simulink model "Fuzzy_and_EKF_tightly"  (R2021b)
settings: Solver=ode4  StartTime=0.0  StopTime=200  FixedStep=1e-2  RelTol=1e-3
values from neighbouring files (symbols this model uses):
  n_J = 0.6    [sensors_model.m]
  n_W = 0.18    [sensors_model.m]
undefined symbols (not defined in the file or in its folder): measure
libraries: fuzblock x1
settings Model: Creator=francescoiotti  LastModifiedBy=pierg
settings ModelReferenceCC: ModelReferenceMinAlgLoopOccurrences=on

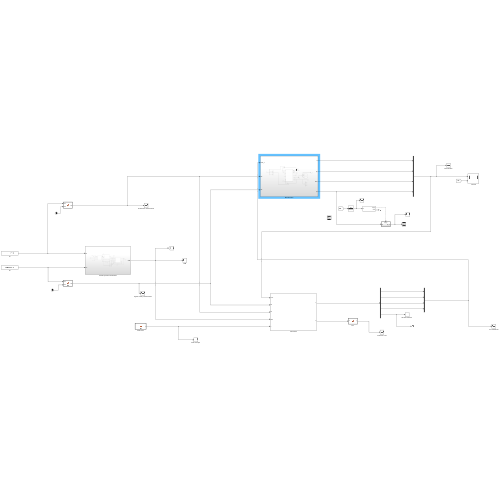
[thumbnail: Simulink's stored preview of the top-level diagram]
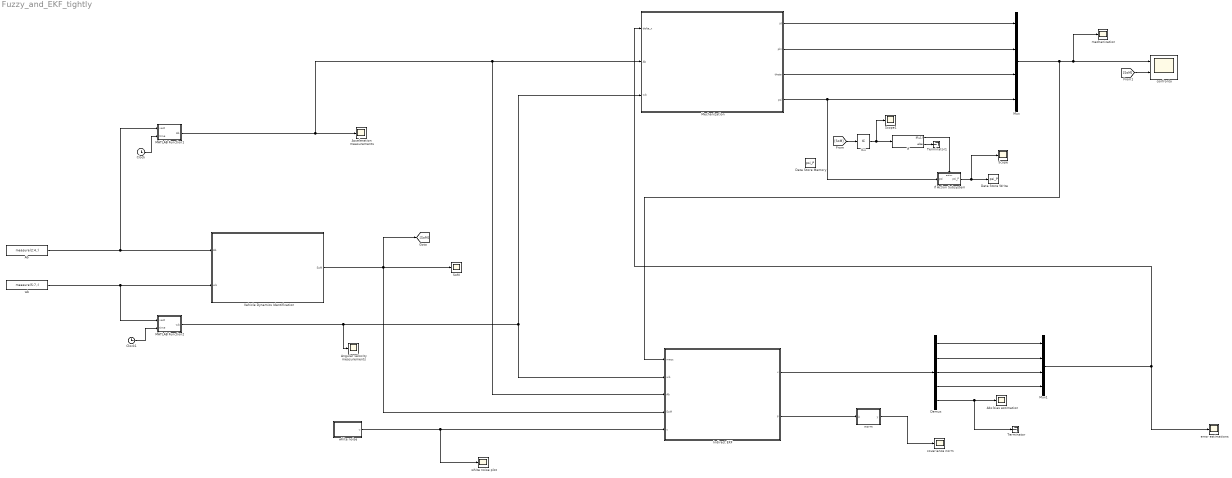
== system Fuzzy_and_EKF_tightly ==
  Ab : Constant  Value=measure(2:4,:)
  Abx bias estimation : Scope
  Acceleration measurements : Scope
  Angular velocity measurements : Scope
  Clock : Clock
  Clock1 : Clock
  Data Store Memory : DataStoreMemory  DataStoreName=psi_P  ReadBeforeWriteMsg=warning  WriteAfterWriteMsg=warning  WriteAfterReadMsg=warning  InitialValue=pi/2  ShowAdditionalParam=off
  Data Store Write : DataStoreWrite  DataStoreName=psi_P  IndexOptions=Index vector (dialog)  Indices=1  OutputSizes=1
  Demux : Demux  Outputs=5
  IC1 : InitialCondition
  If : If  IfExpression=u1
  If Action Subsystem : Subsystem  TreatAsAtomicUnit=on
  Indirect EKF : Subsystem
  MATLAB Function1 : MATLAB Function  TreatAsAtomicUnit=on
  MATLAB Function2 : MATLAB Function  TreatAsAtomicUnit=on
  Mechanization : Subsystem
  Mux : Mux
  Mux1 : Mux
  Scope : Scope
  Scope1 : Scope
  SoM : Scope
  Terminator : Terminator
  Terminator1 : Terminator
  Vehicle Dynamics Identification : Subsystem
  confronto : Scope  NumInputPorts=2
  covariance norm : Scope
  error estimations : Scope
  mechanization : Scope
  norm : MATLAB Function  TreatAsAtomicUnit=on
  wb : Constant  Value=measure(5:7,:)
  white noise : MATLAB Function  TreatAsAtomicUnit=on
  white noise plot : Scope
  wires:
  Vehicle Dynamics Identification/1(SoM) -> SoM/1, [SoM], Indirect EKF/4(SoM)
  Ab/1 -> MATLAB Function1/1(vect), Vehicle Dynamics Identification/1(Ab)
  Indirect EKF/2(P) -> norm/1(A)
  white noise/1(u) -> white noise plot/1, Indirect EKF/5(u)
  norm/1(y) -> covariance norm/1
  MATLAB Function1/1(Ab) -> Acceleration measurements/1, Indirect EKF/3(Ab), Mechanization/2(Ab)
  wb/1 -> MATLAB Function2/1(vect), Vehicle Dynamics Identification/2(wb)
  MATLAB Function2/1(wb) -> Angular velocity measurements/1, Mechanization/3(wb), Indirect EKF/2(wb)
  Clock/1 -> MATLAB Function1/2(time)
  Clock1/1 -> MATLAB Function2/2(time)
  Mux/1 -> confronto/1, mechanization/1, Indirect EKF/1(mecc)
  Mechanization/1(Vf) -> Mux/1
  Mechanization/2(phi) -> Mux/2
  Mechanization/3(theta) -> Mux/3
  Indirect EKF/1(x) -> Demux/1
  Demux/1 -> Mux1/1
  Demux/2 -> Mux1/2
  Demux/3 -> Mux1/3
  Demux/4 -> Mux1/4
  Mux1/1 -> Mechanization/1(delta_x), error estimations/1
  Demux/5 -> Abx bias estimation/1, Terminator/1
  If/1 -> If Action Subsystem/Action
  If Action Subsystem/1(psi_P) -> Scope/1, Data Store Write/1
  If/2 -> Terminator1/1
  [SoM] -> confronto/2
  Mechanization/4(psi) -> Mux/4, If Action Subsystem/1(psi)
  [SoM] -> IC1/1
  IC1/1 -> Scope1/1, If/1

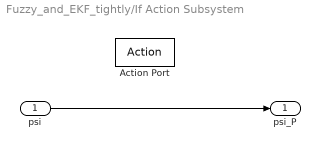
== system Fuzzy_and_EKF_tightly/If Action Subsystem ==
  psi : Inport
  Action Port : ActionPort  ActionPortLabel=if(u1)
  psi_P : Outport
  wires:
  psi/1 -> psi_P/1

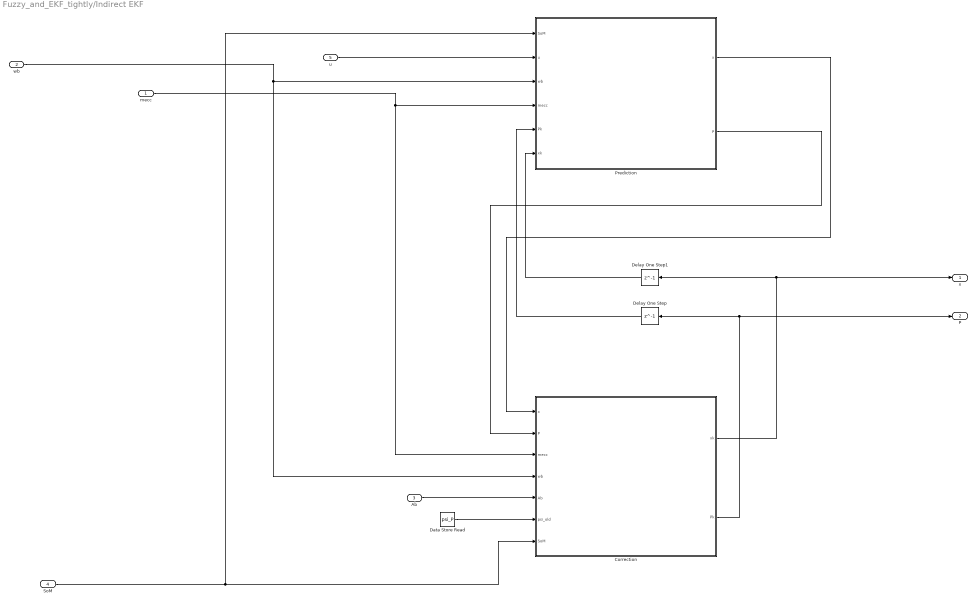
== system Fuzzy_and_EKF_tightly/Indirect EKF ==
  mecc : Inport
  wb : Inport  Port=2
  Ab : Inport  Port=3
  SoM : Inport  Port=4
  u : Inport  Port=5
  Correction : MATLAB Function  TreatAsAtomicUnit=on
  Data Store Read : DataStoreRead  DataStoreName=psi_P  IndexOptions=Index vector (dialog)  Indices=1  OutputSizes=1
  Delay One Step : Delay  DelayLength=1  InitialCondition=eye(5)
  Delay One Step1 : Delay  DelayLength=1  InitialCondition=[0 0 0 0 0]'
  Prediction : MATLAB Function  TreatAsAtomicUnit=on
  x : Outport
  P : Outport  Port=2
  wires:
  Prediction/1(x) -> Correction/1(x)
  Correction/1(xk) -> Delay One Step1/1, x/1
  Correction/2(Pk) -> Delay One Step/1, P/1
  Prediction/2(P) -> Correction/2(P)
  Delay One Step/1 -> Prediction/5(Pk)
  Delay One Step1/1 -> Prediction/6(xk)
  u/1 -> Prediction/2(u)
  wb/1 -> Correction/4(wb), Prediction/3(wb)
  Ab/1 -> Correction/5(Ab)
  mecc/1 -> Correction/3(mecc), Prediction/4(mecc)
  Data Store Read/1 -> Correction/6(psi_old)
  SoM/1 -> Correction/7(SoM), Prediction/1(SoM)

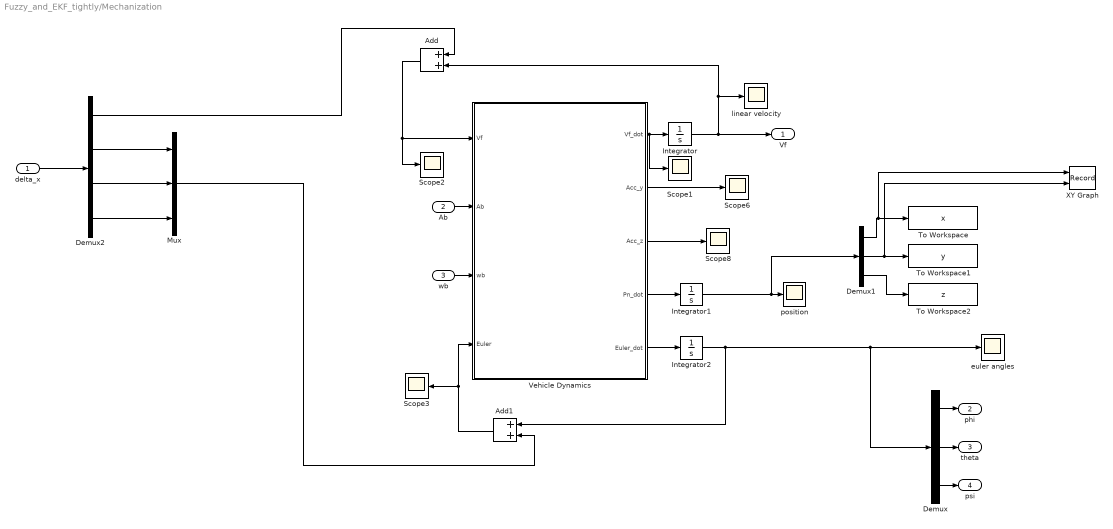
== system Fuzzy_and_EKF_tightly/Mechanization ==
  delta_x : Inport
  Ab : Inport  Port=2
  wb : Inport  Port=3
  Add : Sum
  Add1 : Sum
  Demux : Demux  Outputs=3
  Demux1 : Demux  Outputs=3
  Demux2 : Demux
  Integrator : Integrator
  Integrator1 : Integrator  InitialCondition=[0 0 0]'
  Integrator2 : Integrator  InitialCondition=[0 0 pi/2]'
  Mux : Mux  Inputs=3
  Scope{1..3,6,8} (5 alike) : Scope
  To Workspace : ToWorkspace  VariableName=x  SaveFormat=Structure  SampleTime=-1
  To Workspace1 : ToWorkspace  VariableName=y  SaveFormat=Structure  SampleTime=-1
  To Workspace2 : ToWorkspace  VariableName=z  SaveFormat=Structure  SampleTime=-1
  Vehicle Dynamics : MATLAB Function  TreatAsAtomicUnit=on
  XY Graph : Record  FileSettingsInternal="{\"entries\":[{\"content\":{\"excelSettings\":{\"content\":{},\"type\":\"Streamout.ExcelSettings\"}},\"type\":\"Streamout.FileSettingStorage\",\"uuid\":\"3c158775-b6e3-428c-9659-72c20ea76644\"}],\"packageUris\":[\"http://schema.mathworks.com/mf0/streamout_blocks/R2020a\"],\"version\":\"1.0\"}"  Layout=[1 1]  SignalsInternal="{\"entries\":[{\"content\":{\"signals\":[{\"content\":{\"blockPath\":[\"Fuzzy_and_EKF_tightly/Mechanization/XY Graph\"],\"channel\":[],\"dimensions\":[1,1],\"domain\":\"Fuzzy_and_EKF_tightly/Mechanization/XY Graph\",\"lineColor\":\"#edb120\",\"plots\":[],\"port\":1,\"sid\":[\"\"],\"signalID\":16325,\"signalName\":\"Demux1:1\"},\"type\":\"RecordBlkView.Signal\",\"uuid\":\"bfe6afe1-6902-4355-a286-55c02540e738\"},{\"content\":{\"blockPath\":[\"Fuzzy_and_EKF_tightly/Mechanization/XY Graph\"],\"channel\":[],\"dimensions\":[1,1],\"domain\":\"Fuzzy_and_EKF_tightly/Mechanization/XY Graph\",\"lineColor\":\"#7e2f8e\",\"plots\":[],\"port\":2,\"sid\":[\"\"],\"signalID\":16329,\"signalName\":\"Demux1:2\"},\"type\":\"RecordBlkView.Signal\",\"uuid\":\"bf2d8db9-6f53-45fd-a215-5a4437fe8068\"}]},\"type\":\"RecordBlkView.InputSignals\",\"uuid\":\"d2e0fcf7-0ff7-4170-9add-71b356b071cf\"}],\"packageUris\":[\"http://schema.mathworks.com/mf0/streamout_blocks/R2020a\"],\"version\":\"1.0\"}"  VisualizationBindings="{\"xyplotplugin\":{\"info\":[{\"series\":[],\"subplotID\":1}]}}"  CompatibilityTag=XY
  euler angles : Scope
  linear velocity : Scope
  position : Scope
  Vf : Outport
  phi : Outport  Port=2
  theta : Outport  Port=3
  psi : Outport  Port=4
  wires:
  Integrator/1 -> Vf/1, Add/2, linear velocity/1
  Vehicle Dynamics/3(Acc_z) -> Scope8/1
  Vehicle Dynamics/1(Vf_dot) -> Scope1/1, Integrator/1
  wb/1 -> Vehicle Dynamics/3(wb)
  Vehicle Dynamics/4(Pn_dot) -> Integrator1/1
  Vehicle Dynamics/2(Acc_y) -> Scope6/1
  Integrator1/1 -> Demux1/1, position/1
  Vehicle Dynamics/5(Euler_dot) -> Integrator2/1
  Demux/2 -> theta/1
  Demux/3 -> psi/1
  Demux/1 -> phi/1
  Ab/1 -> Vehicle Dynamics/2(Ab)
  Demux1/1 -> XY Graph/1, To Workspace/1
  Demux1/2 -> XY Graph/2, To Workspace1/1
  Demux1/3 -> To Workspace2/1
  Integrator2/1 -> Add1/1, Demux/1, euler angles/1
  delta_x/1 -> Demux2/1
  Demux2/2 -> Mux/1
  Demux2/3 -> Mux/2
  Demux2/4 -> Mux/3
  Mux/1 -> Add1/2
  Add1/1 -> Scope3/1, Vehicle Dynamics/4(Euler)
  Demux2/1 -> Add/1
  Add/1 -> Scope2/1, Vehicle Dynamics/1(Vf)

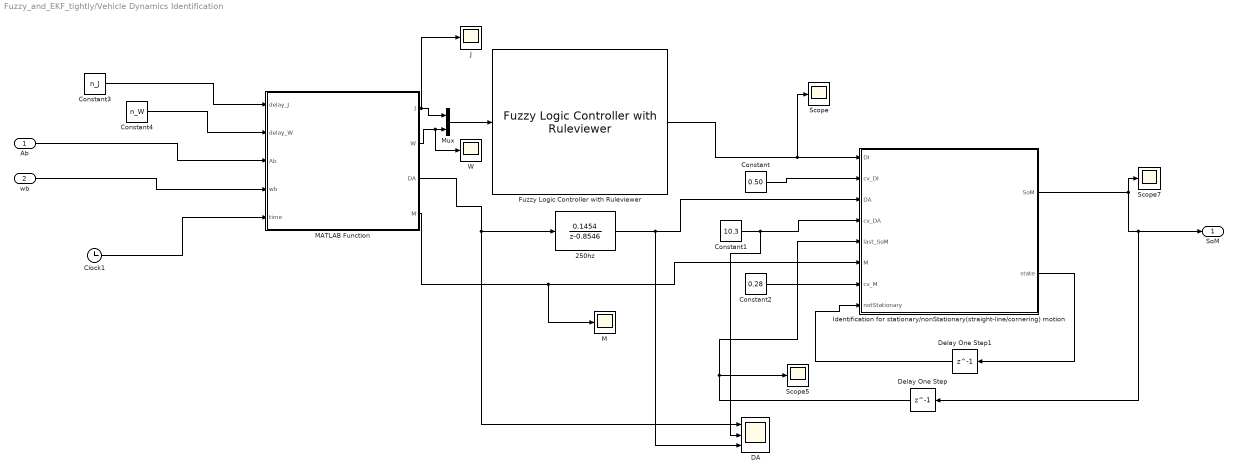
== system Fuzzy_and_EKF_tightly/Vehicle Dynamics Identification ==
  Ab : Inport
  wb : Inport  Port=2
  250hz : DiscreteTransferFcn  Numerator=[0.1454]  Denominator=[1 -0.8546]
  Clock1 : Clock
  Constant : Constant  Value=0.50
  Constant1 : Constant  Value=10.3
  Constant2 : Constant  Value=0.28
  Constant3 : Constant  Value=n_J
  Constant4 : Constant  Value=n_W
  DA : Scope  NumInputPorts=3
  Delay One Step : Delay  DelayLength=1  InitialCondition=0
  Delay One Step1 : Delay  DelayLength=1  InitialCondition=0
  Fuzzy Logic Controller with Ruleviewer : fuzblock/Fuzzy Logic  Controller  with Ruleviewer  fismatrix=pippo  Ts=10
  Identification for stationary/nonStationary(straight-line/cornering) motion : MATLAB Function  TreatAsAtomicUnit=on
  J : Scope
  M : Scope
  MATLAB Function : MATLAB Function  TreatAsAtomicUnit=on
  Mux : Mux  Inputs=2
  Scope : Scope
  Scope5 : Scope
  Scope7 : Scope
  W : Scope
  SoM : Outport
  wires:
  Constant1/1 -> DA/2, Identification for stationary/nonStationary(straight-line/cornering) motion/4(cv_DA)
  MATLAB Function/3(DA) -> 250hz/1, DA/1
  MATLAB Function/1(J) -> J/1, Mux/1
  Fuzzy Logic Controller with Ruleviewer/1 -> Scope/1, Identification for stationary/nonStationary(straight-line/cornering) motion/1(DI)
  MATLAB Function/4(M) -> M/1, Identification for stationary/nonStationary(straight-line/cornering) motion/6(M)
  Identification for stationary/nonStationary(straight-line/cornering) motion/1(SoM) -> SoM/1, Delay One Step/1, Scope7/1
  Constant2/1 -> Identification for stationary/nonStationary(straight-line/cornering) motion/7(cv_M)
  Constant/1 -> Identification for stationary/nonStationary(straight-line/cornering) motion/2(cv_DI)
  MATLAB Function/2(W) -> W/1, Mux/2
  Mux/1 -> Fuzzy Logic Controller with Ruleviewer/1
  Clock1/1 -> MATLAB Function/5(time)
  wb/1 -> MATLAB Function/4(wb)
  Ab/1 -> MATLAB Function/3(Ab)
  Constant3/1 -> MATLAB Function/1(delay_J)
  Delay One Step/1 -> Scope5/1, Identification for stationary/nonStationary(straight-line/cornering) motion/5(last_SoM)
  Identification for stationary/nonStationary(straight-line/cornering) motion/2(state) -> Delay One Step1/1
  Delay One Step1/1 -> Identification for stationary/nonStationary(straight-line/cornering) motion/8(notStationary)
  250hz/1 -> DA/3, Identification for stationary/nonStationary(straight-line/cornering) motion/3(DA)
  Constant4/1 -> MATLAB Function/2(delay_W)

== matlab function Fuzzy_and_EKF_tightly/MATLAB Function2 ==
  data: vect input; time input; wb output
function wb = fcn(vect, time)
t = int64(time/1e-2)+1;
wb = vect(:,t);

== matlab function Fuzzy_and_EKF_tightly/Mechanization/Vehicle Dynamics ==
  data: Vf input; Ab input; wb input; Euler input; Vf_dot output; Acc_y output; Acc_z output; Pn_dot output; Euler_dot output
function [Vf_dot, Acc_y, Acc_z, Pn_dot, Euler_dot] = Vehicle_model(Vf, Ab, wb, Euler)
%% Land Vehicle Dynamic model
% x_dot is the derivative of x

Abx = Ab(1);
Aby = Ab(2);
Abz = Ab(3);

wbx = wb(1);
wby = wb(2);
wbz = wb(3);

% Euler angles
phi = Euler(1);
theta = Euler(2);
psi = Euler(3);

% Constant
g = 9.81;

% Model
Vf_dot = Abx - g*sin(theta);
Acc_y = Aby + g*sin(phi)*cos(theta);
Acc_z = -Abz - g*cos(phi)*cos(theta);
phi_dot = wbx + sin(phi)*tan(theta)*wby + cos(phi)*tan(theta)*wbz;
theta_dot = cos(phi)*wby - sin(phi)*wbz;
psi_dot = wby*sin(phi)/cos(theta) + cos(phi)/cos(theta) * wbz;
Pnn_dot = Vf*cos(theta)*cos(psi);
Pne_dot = Vf*cos(theta)*sin(psi);
Pnd_dot = Vf*sin(theta);

Ab = [Abx, Aby, Abz]';
Euler_dot = [phi_dot, theta_dot, psi_dot]';
Pn_dot = [Pnn_dot, Pne_dot, Pnd_dot]';

== matlab function Fuzzy_and_EKF_tightly/Vehicle Dynamics Identification/Identification for stationary//nonStationary(straight-line//cornering) motion ==
  data: DI input; cv_DI input; DA input; cv_DA input; last_SoM input; M input; SoM output; cv_M input; notStationary input; state output
function [SoM, state] = type_of_motion_decision_loop(DI, cv_DI, DA, cv_DA, last_SoM, M, cv_M, notStationary)

    %% Identification for stationary/nonStationary(straight-line/cornering) motion
    % SoM : state of motion for landend vehicle
    % last_SoM: previous state of motion for landend vehicle
    % 0 := Stationary
    % 1 := straight-line motion
    % 2 := cornering motion
    % notStationary: if 1 the vehicle is not stationary

    SoM = 0;

    if last_SoM == 0 && DA > cv_DA      
        notStationary = 1;
    elseif	last_SoM && DA < cv_DA && DI < cv_DI
        SoM = 0;
        notStationary = 0;
    else 
        SoM = last_SoM;
%         notStationary = 0;
    end
    
    %Run this only if notStactionary
    if notStationary
        SoM = last_SoM;
    end

    if notStationary && (M >= cv_M)
        SoM = 2;
    end

    if notStationary && (M < cv_M)
        SoM = 1;
    end

    state = notStationary;

== matlab function Fuzzy_and_EKF_tightly/Vehicle Dynamics Identification/MATLAB Function ==
  data: delay_J input; delay_W input; Ab input; J output; wb input; time input; W output; DA output; M output
function [J, W, DA, M] = functional_computation(delay_J, delay_W, Ab, wb, time)
% Trasformo i tempi in passi
n_J = int64(delay_J/1e-2);
n_W = int64(delay_W/1e-2);
t = int64(time/1e-2);
p = int64(2.5/1e-2);
m = int64(1/1e-2);
% Inizializzo i funzionali
J = 0;
W = 0;
DA = 0;
Mwbz = 0;

% Calcolo J
for i=t-n_J:t
%   Controllo nel caso in cui t < n ed escludo i termini con indici
%   negativi
    if i > 1
        J = J + abs( norm(Ab(:,i)) - norm(Ab(:,i-1)) );
    end
end

% Calcolo W
for i=t-n_W:t
%   Controllo nel caso in cui t < n ed escludo i termini con indici
%   negativi
    if i > 0
        W = W + abs( sqrt(wb(1,i)^2 + wb(2,i)^2) ); % / double(n);
    end
end


% Calcolo DA
for i=t-p:t
%   Controllo nel caso in cui t < n ed escludo i termini con indici
%   negativi
    if t-p > 0
        DA = DA + abs( Ab(1,i) - Ab(1,t-p) );
    end
end


% Calcolo M
for i=t-m:t
%   Controllo nel caso in cui t < n ed escludo i termini con indici
%   negativi
    if i > 1
        Mwbz = Mwbz + abs(wb(3,i));
    end
end
M = Mwbz / double(m);

== matlab function Fuzzy_and_EKF_tightly/Indirect EKF/Prediction ==
  data: SoM input; u input; wb input; mecc input; Pk input; x output; xk input; P output
function [x, P] = prediction(SoM, u, wb, mecc, Pk, xk)

% Estraggo le componenti di velocità angolare
wbx = wb(1);
wby = wb(2);
wbz = wb(3);

% Estraggo le grandezze calcolate con la meccanizzazione
Vf = mecc(1);
phi = mecc(2);
theta = mecc(3);
psi = mecc(4);

% Costante
g = 9.81;

% Definisco gli elementi della matrice F
f13 = -g*cos(theta);
f22 = cos(phi)*tan(theta)*wby - sin(phi)*tan(theta)*wbz;
f23 = sin(phi)*wby*sec(theta)^2 + cos(phi)*wbz*sec(theta)^2;
f32 = -sin(phi)*wby - cos(phi)*wbz;
f42 = cos(phi)*wby*sec(theta) - sin(phi)*wbz*sec(theta);
f43 = sin(phi)*tan(theta)*wby*sec(theta) + cos(phi)*tan(theta)*wbz*sec(theta);

F = [0  0  f13  0  1;
     0 f22 f23  0  0;
     0 f32  0   0  0;
     0 f42 f43  0  0;
     0  0   0   0  0;];

% Definisco gli elementi della matrice G
g23 = sin(phi)*tan(theta);
g24 = cos(phi)*tan(theta);
g33 = cos(phi);
g34 = -sin(phi);
g43 = sin(phi)*sec(theta);
g44 = cos(phi)*sec(theta);

G = [1  0  0   0  0;
     0  1 g23 g24 0;
     0  0 g33 g34 0;
     0  0 g43 g44 0;
     0  0  0   0  1;];

% Formula di predizione dello stato
% if SoM == 0
%     x = [xk(1) xk(2) xk(3) xk(4) 0]';
% elseif SoM == 1
%     x = [0 xk(2) 0 0 0]';
% elseif SoM == 2
%     x = [xk(1) 0 0 0 0]';
% else
%     x = xk;
% end
x = zeros(5,1);


% Definisco la matrice di covarianza del rumore di processo Q
qAbx = 0.001; % densità spettrale
qwbx = 0.5; %0.1;
qwby = 0.1;
qwbz = 0.1;
qb = 0;
Q = diag([qAbx, qwbx, qwby, qwbz, qb]);

% Formula di predizione della covarianza
P = F*Pk*F' + G*Q*G';

== matlab function Fuzzy_and_EKF_tightly/Indirect EKF/Correction ==
  data: x input; xk output size=[5 1]; P input; mecc input; wb input; Ab input; psi_old input; Pk output size=[5 5]; SoM input
function [xk, Pk] = correction(x, P, mecc, wb, Ab, psi_old, SoM)
% Estraggo le componenti di accelerazione
Abx = Ab(1);
Aby = Ab(2);
Abz = Ab(3);

% Estraggo le componenti di velocità angolare
wbx = wb(1);
wby = wb(2);
wbz = wb(3);

% Estraggo le grandezze calcolate con la meccanizzazione
Vf = mecc(1);
phi = mecc(2);
theta = mecc(3);
psi = mecc(4);

% Costante
g = 9.81;

% z = [ Vf ; phi-phi_a ; theta-theta_a ; psi-psi_p ]
if SoM == 0

    % Definisco la matrice H
    H = [ 1 0 0 0 0;
          0 1 0 0 0;
          0 0 1 0 0;
          0 0 0 1 0;];
    % Deviazioni standard rumori di misura in fase stazionaria
    sigma_deltaVf_ZUPT = 0.02;
    sigma_deltaPhi = 0.2;
    sigma_deltaTheta = 0.2;
    sigma_deltaPsi = 0.02;
    % Matrice di covarianza
    R = diag([sigma_deltaVf_ZUPT^2, sigma_deltaPhi^2, sigma_deltaTheta^2, sigma_deltaPsi^2]);

    % Misure dynamics-derived
    phi_A = asin(-Aby / sqrt(g^2 - Abx^2));
    theta_A = asin(Abx/g);
    psi_P = psi_old;

    z = [Vf; phi - phi_A; theta - theta_A; psi - psi_P];

elseif SoM == 1

    % Definisco la matrice H
    H = [0 1 0 0 0];

    % Deviazioni standard rumori di misura in fase di movimento lineare
    sigma_deltaPhi = 0.2;
    % Matrice di covarianza
    R = sigma_deltaPhi^2;
    
    % Misure dynamics-derived
    phi_A = asin(-Aby / sqrt(g^2 - Abx^2));

    z = phi - phi_A;

elseif SoM == 2

    % Definisco la matrice H
    H = [1 0 0 0 0];

    % Deviazioni standard rumori di misura in fase di cornering
    sigma_deltaVf_C = 0.02;
    % Matrice di covarianza
    R = sigma_deltaVf_C^2;
    
    % Misure dynamics-derived
    Vf_C = (Aby + g*sin(phi)*cos(theta)) / wbz;

    z = Vf - Vf_C;

else
%   Caso unaided
    H = zeros(4,5);
    R = eye(4);
    z = zeros(4,1);
    fprintf('SoM non si identifica in un genere');

end

% Innovazione
e = z - H * x;
% Covarianza dell'innovazione
S = H * P * H' + R;
L = P * H' * S^(-1);
% Correzione
xk = x + L*e;
% Pk = (eye(5) - L*H) * P * (eye(5) - L*H)' + L*R*L';
Pk = (eye(5) - L*H) * P;

== matlab function Fuzzy_and_EKF_tightly/white noise ==
  data: u output
function u = fcn()
% Accelerometer 
stdv_a = 0.0055; % standard deviation
Wna = stdv_a*randn(1,1); % White Noise
% Gyroscope
stdv_g = 0.6325; % standard deviation
Wng = stdv_g*randn(1,3); % White Noise

u = [Wna, Wng, 0]';

== matlab function Fuzzy_and_EKF_tightly/norm ==
  data: A input; y output
function y = fcn(A)
y = norm(A);

== matlab function Fuzzy_and_EKF_tightly/MATLAB Function1 ==
  data: vect input; Ab output; time input
function Ab = fcn(vect, time)
t = int64(time/1e-2)+1;
Ab = vect(:,t);
